simulink model "Rot_Pen_LQR"  (R2017a)
settings: Solver=VariableStepAuto  StartTime=0.0  StopTime=10.0  RelTol=1e-3
values from neighbouring files (symbols this model uses):
  A = [[0 , 0 , 1 , 0] ... (first row only)    [RotPen.m]
  B = [0 ; 0 ; Kt*(Jp+Mp*lp^2)/Rm/(Jeq*Jp+Jeq*Mp*lp^2+Mp*r^2*Jp) ; Mp*lp*Kt*r/Rm/(Jeq*Jp+Jeq*Mp*lp^2+Mp*r^2*Jp)]    [RotPen.m]
  C = [[1 0 0 0] ... (first row only)    [RotPen.m]
  D = [0 ; 0 ; 0 ; 0]    [RotPen.m]
  IC = [0 0.2 0 0]    [RotPen.m]
undefined symbols (not defined in the file or in its folder): K
settings Model: Creator=Fouad  LastModifiedBy=Fouad

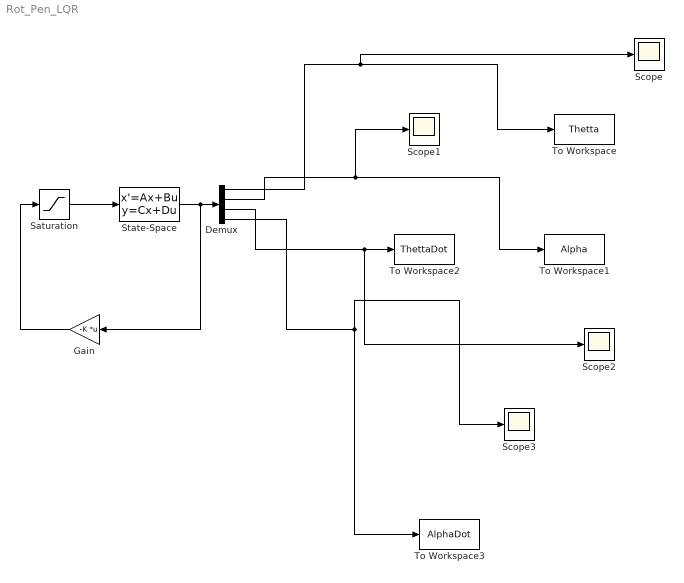
== system Rot_Pen_LQR ==
  Demux : Demux
  Gain : Gain  Gain=-K  Multiplication=Matrix(K*u)
  Saturation : Saturate  UpperLimit=18  LowerLimit=-18
  Scope{,1..3} (4 alike) : Scope
  State-Space : StateSpace  A=A  B=B  C=C  D=D  X0=IC
  To Workspace : ToWorkspace  VariableName=Thetta  SampleTime=0.01
  To Workspace1 : ToWorkspace  VariableName=Alpha  SampleTime=0.01
  To Workspace2 : ToWorkspace  VariableName=ThettaDot  SampleTime=0.01
  To Workspace3 : ToWorkspace  VariableName=AlphaDot  SampleTime=0.01
  wires:
  State-Space/1 -> Gain/1, Demux/1
  Demux/1 -> Scope/1, To Workspace/1
  Demux/2 -> Scope1/1, To Workspace1/1
  Demux/3 -> Scope2/1, To Workspace2/1
  Demux/4 -> Scope3/1, To Workspace3/1
  Saturation/1 -> State-Space/1
  Gain/1 -> Saturation/1
